simulink model "PIL_NO_RPI"  (R2021a)
settings: Solver=FixedStepAuto  StartTime=0.0  StopTime=50  FixedStep=0.001  RelTol=1e-3  EnableMultiTasking=on
undefined symbols (not defined in the file or in its folder): act_dmp, act_omega, Actuator, Aerodynamics, aMode, Autopilot, c_b_WGS, c_be, c_flat, c_grav, c_h_geop0, c_h_geope, c_pa0, c_pe, c_r0, c_rot, c_rsma, c_Tmp0, d_siB_0, d_siB_max, d_siB_min, dd_siB_max, dd_siB_min, DiscIntNeverNeededParam, e_pa, e_Tmp, fin_maxrate, flag_I_act_switch, flag_I_aero_switch, flag_I_flat, flag_I_gravity_switch, flag_I_rot, hcr, HIL_Data, JMMM_0, JMMM_e, JSPB_e, lat_0, lon_0, Mass_Props, mB_0, mM_0, mM_e, p, pBII_0, phi, pMPB, pNPB, propellant_kg, prp_FBPB, prp_mdot, prp_T, psi, pSPB, q, qEG_0, qIB_0, qIE_0, r, sgc ... (+28)
libraries: simulink x46, simulink_extras x10, aerolibcommonsys x4
(part 1 of 21)
settings Model: SimulationMode=external  CodeVerificationMode=processor-in-the-loop (pil)  ExtModeTrigDuration=10  Creator=m.hiepp  LastModifiedBy=benme
settings SolverCC: AlgebraicLoopSolver=TrustRegion  PositivePriorityOrder=on  AutoInsertRateTranBlk=on
settings DataIOCC: SignalLogging=off  ReturnWorkspaceOutputs=off
settings OptimizationCC: EnhancedBackFolding=on  PassReuseOutputArgsAs=Individual arguments  ZeroExternalMemoryAtStartup=off  ZeroInternalMemoryAtStartup=off  MaxStackSize=64  OptimizeBlockOrder=speed  DifferentSizesBufferReuse=on  OptimizationCustomize=off  EfficientTunableParamExpr=on
settings DebuggingCC: ParameterPrecisionLossMsg=none  ParameterTunabilityLossMsg=error  SFMachineParentedDataDiag=warning  UnderSpecifiedDimensionMsg=warning  ArithmeticOperatorsInVariantConditions=warning
settings HardwareCC: ProdBitPerPointer=32  ProdBitPerSizeT=32  ProdBitPerPtrDiffT=32  ProdLargestAtomicInteger=Long  ProdLargestAtomicFloat=Double  ProdWordSize=32  ProdLongLongMode=on  ProdHWDeviceType=ARM Compatible->ARM Cortex
settings SFSimCC: MATLABDynamicMemAlloc=off  CustomCodeUndefinedFunction=UseInterfaceOnly  SimTargetLang=C++
settings RTWCC: SystemTargetFile=ert.tlc  HardwareBoard=PX4 Pixhawk 2.1 (Cube)  TLCOptions="-aInlineSetEventsForThisBaseRateFcn=TLC_FALSE -aSuppressMultiTaskScheduler=TLC_FALSE  -aRateBasedStepFcn=0"  TemplateMakefile=ert_default_tmf  GenerateReport=on  Toolchain=GNU Tools for PX4 Autopilots  IncludeHyperlinkInReport=on  LaunchReport=on  PortableWordSizes=on  CreateSILPILBlock=PIL  TargetLang=C++  GenerateTraceInfo=on  GenerateTraceReport=on  GenerateTraceReportSl=on  GenerateTraceReportSf=on  GenerateTraceReportEml=on
settings CodeAppCC: ForceParamTrailComments=on  IgnoreCustomStorageClasses=off  MaxIdLength=95  OperatorAnnotations=on  SimulinkDataObjDesc=on  SFDataObjDesc=on  InsertBlockDesc=on
settings ERTTargetCC: SupportContinuousTime=on  ExtModeTransport=3  ExtModeStaticAlloc=on  ExtModeStaticAllocSize=1024  ExtModeMexFile=ext_xcp  ExtModeIntrfLevel=Level2 - Open

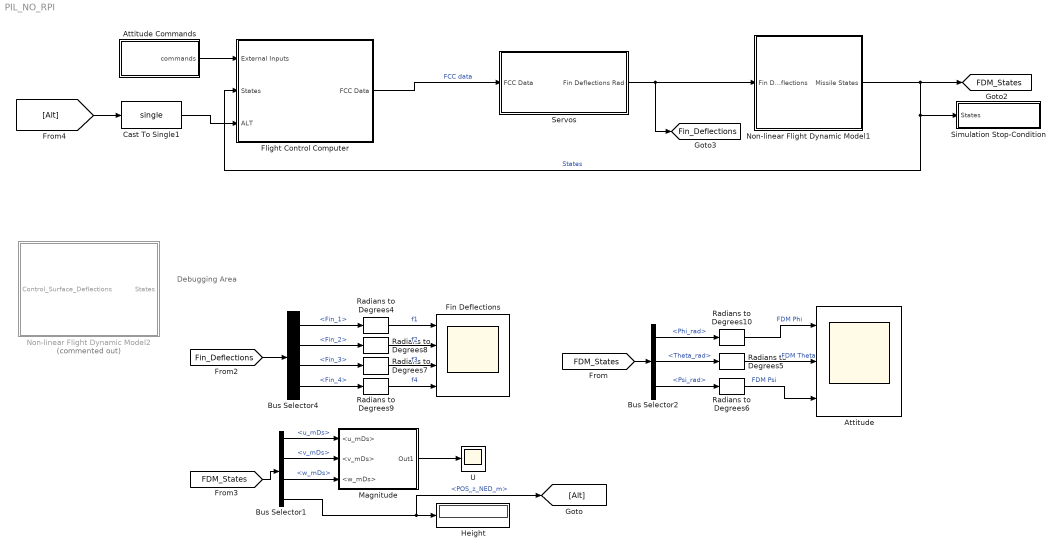
== system PIL_NO_RPI ==
  note: Debugging Area
  Attitude : Scope  NumInputPorts=3
  Attitude Commands : Subsystem
  Bus Selector1 : BusSelector  OutputSignals=Translation_States.u_mDs,Translation_States.v_mDs,Translation_States.w_mDs,POS_NED.POS_z_NED_m
  Bus Selector2 : BusSelector  OutputSignals=Attitude_States.ATT_Euler.Phi_rad,Attitude_States.ATT_Euler.Theta_rad,Attitude_States.ATT_Euler.Psi_rad
  Bus Selector4 : BusSelector  OutputSignals=Fin_1,Fin_2,Fin_3,Fin_4
  Cast To Single1 : DataTypeConversion  OutDataTypeStr=single
  Fin Deflections : Scope  NumInputPorts=4
  Flight Control Computer : Subsystem  VariantControl=VSS_FCC_REAL
  Height : Display
  Magnitude : Subsystem
  Non-linear Flight Dynamic Model1 : Subsystem  VariantControl=VSS_FDM_SOPH
      mask init:
      | load('generated_FDM_params')
  Non-linear Flight Dynamic Model2 : Subsystem  Commented=on  VariantControl=VSS_FDM_SOPH
      mask init:
      | load('generated_FDM_params')
  Radians to Degrees{4..10} (7 alike) : simulink_extras/Transformations/Radians to Degrees
  Servos : Subsystem  VariantControl=VSS_SERVOS_OFF
  Simulation Stop-Condition : Subsystem
  U : Scope
  tag scope: FDM_States=global, Fin_Deflections=global
  wires:
  Bus Selector2/3 -> Radians to Degrees6/1  "<Psi_rad>"
  Bus Selector4/2 -> Radians to Degrees8/1  "<Fin_2>"
  Bus Selector2/2 -> Radians to Degrees5/1  "<Theta_rad>"
  Radians to Degrees9/1 -> Fin Deflections/4  "f4"
  Radians to Degrees7/1 -> Fin Deflections/3  "f3"
  Radians to Degrees8/1 -> Fin Deflections/2  "f2"
  Bus Selector2/1 -> Radians to Degrees10/1  "<Phi_rad>"
  Servos/1(Fin Deflections Rad) -> Non-linear Flight Dynamic Model1/1(Fin Deflections), [Fin_Deflections]
  Bus Selector4/1 -> Radians to Degrees4/1  "<Fin_1>"
  [Fin_Deflections] -> Bus Selector4/1
  Attitude Commands/1(commands) -> Flight Control Computer/1(External Inputs)
  Radians to Degrees5/1 -> Attitude/2  "FDM Theta"
  [FDM_States] -> Bus Selector2/1
  Non-linear Flight Dynamic Model1/1(Missile States) -> Flight Control Computer/2(States), Simulation Stop-Condition/1(States), [FDM_States]  "States"
  Bus Selector4/3 -> Radians to Degrees7/1  "<Fin_3>"
  Radians to Degrees4/1 -> Fin Deflections/1  "f1"
  Radians to Degrees10/1 -> Attitude/1  "FDM Phi"
  Bus Selector4/4 -> Radians to Degrees9/1  "<Fin_4>"
  Radians to Degrees6/1 -> Attitude/3  "FDM Psi"
  Flight Control Computer/1(FCC Data) -> Servos/1(FCC Data)  "FCC data"
  [FDM_States] -> Bus Selector1/1
  Bus Selector1/4 -> [Alt], Height/1  "<POS_z_NED_m>"
  Bus Selector1/1 -> Magnitude/1(<u_mDs>)  "<u_mDs>"
  Bus Selector1/2 -> Magnitude/2(<v_mDs>)  "<v_mDs>"
  Bus Selector1/3 -> Magnitude/3(<w_mDs>)  "<w_mDs>"
  Magnitude/1(Out1) -> U/1
  Cast To Single1/1 -> Flight Control Computer/3("ALT ")
  [Alt] -> Cast To Single1/1

== system PIL_NO_RPI/Attitude Commands ==
  Bus Creator : BusCreator  Inputs=3
  Zero : Constant  Value=0  OutDataTypeStr=Inherit: Inherit via back propagation
  Zero1 : Constant  Value=0  OutDataTypeStr=Inherit: Inherit via back propagation
  Zero2 : Constant  Value=0  OutDataTypeStr=Inherit: Inherit via back propagation
  commands : Outport
  wires:
  Bus Creator/1 -> commands/1
  Zero/1 -> Bus Creator/3  "psi cmd rad"
  Zero1/1 -> Bus Creator/2  "theta cmd rad"
  Zero2/1 -> Bus Creator/1  "phi cmd rad"

== system PIL_NO_RPI/Flight Control Computer ==
  note: State Estimation:
      | 0 - use state variables calculated by FDM.
      | 1 - use or our own INS
  External Inputs : Inport
  States : Inport  Port=2
  "ALT " : Inport  Port=3
  Communication Delay - 7ms : Subsystem
  Communication Delay - 7ms1 : Subsystem
  Communication Delay - 7ms2 : Subsystem
  Constant4 : Constant  OutDataTypeStr=single
  Debug : Scope
  FCC Sync : Scope
  In Sync : Subsystem
  Pixhawk1 : Subsystem  TreatAsAtomicUnit=on  VariantControl=VSS_FCC_EMUL
  Recieve from Pixhawk : Subsystem
  Send to Pixhawk : Subsystem
  FCC Data : Outport
  wires:
  Constant4/1 -> Send to Pixhawk/3(Use FDM States)
  External Inputs/1 -> Send to Pixhawk/2(External_Inputs)
  States/1 -> Send to Pixhawk/1(States)
  Send to Pixhawk/1(Heartbeat Sent) -> In Sync/1(send)
  Recieve from Pixhawk/1(Heartbeat recieved1) -> In Sync/2(receive)  "receive"
  Recieve from Pixhawk/3(Other1) -> Debug/1
  In Sync/1(Heartbeat Sync) -> FCC Sync/1
  Communication Delay - 7ms2/1(Signal Recieved) -> Recieve from Pixhawk/1(data in1)
  Send to Pixhawk/2(data out) -> Communication Delay - 7ms/1(Signal Sent)
  "ALT "/1 -> Communication Delay - 7ms1/1(Signal Sent)
  Recieve from Pixhawk/2(fin_cmd_rad1) -> FCC Data/1
  Communication Delay - 7ms/1(Signal Recieved) -> Pixhawk1/1(Input Data)
  Communication Delay - 7ms1/1(Signal Recieved) -> Pixhawk1/2("ALT ")
  Pixhawk1/1(Output Data) -> Communication Delay - 7ms2/1(Signal Sent)

== system PIL_NO_RPI/Magnitude ==
  <u_mDs> : Inport
  <v_mDs> : Inport  Port=2
  <w_mDs> : Inport  Port=3
  Add1 : Sum  Inputs=+++
  Square Root1 : Sqrt  SaturateOnIntegerOverflow=on
  Square3 : Math  Operator=square  SaturateOnIntegerOverflow=on
  Square4 : Math  Operator=square  SaturateOnIntegerOverflow=on
  Square5 : Math  Operator=square  SaturateOnIntegerOverflow=on
  Out1 : Outport
  wires:
  Add1/1 -> Square Root1/1
  Square4/1 -> Add1/2
  Square5/1 -> Add1/3
  <u_mDs>/1 -> Square3/1
  Square Root1/1 -> Out1/1
  Square3/1 -> Add1/1
  <w_mDs>/1 -> Square5/1
  <v_mDs>/1 -> Square4/1

== system PIL_NO_RPI/Non-linear Flight Dynamic Model1 ==
  Fin Deflections : Inport
  Environment : Subsystem
  Extract States : Subsystem
  GRM_Airframe : Subsystem
      mask Display: image('$imagefile'); % Use "Edit Image" on toolstrip to change.
  Stop-Condition : Subsystem
  Subsystem1 : Subsystem  Commented=on
  Translate Fins : Subsystem
  Missile States : Outport  VectorParamsAs1DForOutWhenUnconnected=off
  wires:
  Fin Deflections/1 -> Translate Fins/1(Servo Deflections)
  Extract States/1(States) -> Missile States/1, Stop-Condition/1(States)  "States"
  Translate Fins/1(afinB) -> GRM_Airframe/1(siB_cmd)
  GRM_Airframe/1(airfr) -> Extract States/1(airfr_bus)
  Environment/1(env_glbl_bus) -> GRM_Airframe/2(T_sim_glbl)

== system PIL_NO_RPI/Non-linear Flight Dynamic Model2 ==
  note: This block is the work of Thomas. Should you have any questions, hes the guy to ask.
  Control_Surface_Deflections : Inport
  Extract Relevant States : Subsystem
  GRM_Airframe : Subsystem
      mask Display: image('$imagefile'); % Use "Edit Image" on toolstrip to change.
  Subsystem1 : Subsystem
  environment_global : Subsystem
  States : Outport  VectorParamsAs1DForOutWhenUnconnected=off
  wires:
  environment_global/1(env_glbl_bus) -> GRM_Airframe/2(T_sim_glbl)
  Subsystem1/1(afinB) -> GRM_Airframe/1(siB_cmd)
  Extract Relevant States/1(States) -> States/1
  Control_Surface_Deflections/1 -> Subsystem1/1(Servo Deflections)
  GRM_Airframe/1(airfr) -> Extract Relevant States/1(airfr_bus)

== system PIL_NO_RPI/Servos ==
  FCC Data : Inport
  Bus Creator : BusCreator  Inputs=4
  Bus Selector : BusSelector  OutputSignals=Fin_1_Cmd_rad,Fin_2_Cmd_rad,Fin_3_Cmd_rad,Fin_4_Cmd_rad
  Gain{,1..3} (4 alike) : Gain
  Transfer Fcn{1..4} (4 alike) : TransferFcn  Numerator=33770  Denominator=[1 395.7 33770]
  Fin Deflections Rad : Outport
  wires:
  FCC Data/1 -> Bus Selector/1
  Bus Selector/1 -> Transfer Fcn1/1  "<Fin_1_Cmd_rad>"
  Bus Selector/2 -> Transfer Fcn2/1  "<Fin_2_Cmd_rad>"
  Bus Selector/3 -> Transfer Fcn3/1  "<Fin_3_Cmd_rad>"
  Bus Selector/4 -> Transfer Fcn4/1  "<Fin_4_Cmd_rad>"
  Transfer Fcn1/1 -> Gain/1  "Fin_1"
  Transfer Fcn2/1 -> Gain1/1  "Fin_2"
  Transfer Fcn3/1 -> Gain2/1  "Fin_3"
  Transfer Fcn4/1 -> Gain3/1  "Fin_4"
  Bus Creator/1 -> Fin Deflections Rad/1
  Gain/1 -> Bus Creator/1  "Fin_1"
  Gain1/1 -> Bus Creator/2  "Fin_2"
  Gain2/1 -> Bus Creator/3  "Fin_3"
  Gain3/1 -> Bus Creator/4  "Fin_4"

== system PIL_NO_RPI/Simulation Stop-Condition ==
  note: Stops the simulation when the rocket hits the ground (Z~0)
  States : Inport
  Bus Selector1 : BusSelector  OutputSignals=POS_NED.POS_z_NED_m
  Compare To Constant : Subsystem  mask(Compare To Constant){relop=>=, const=-10*eps, OutDataTypeStr=boolean, ZeroCross=on}
      mask prompts: relop "Simulink:masks:Operator_MP"; const "Simulink:masks:ConstantValue_MP"; OutDataTypeStr "Simulink:masks:OutputDataType_MP"; ZeroCross "Simulink:masks:EnableZerocrossingDetection_MP"
      mask help: Simulink:masks:CompareToConstant_MD
      mask init:
      | blkName = gcb;
      | 
      | if strcmp(get_param(gcbh,'OutDataTypeStr'),'boolean')
      | 	setValue = 'boolean';
      | else
      | 	setValue = 'fixdt(0, 8)';
      | end
      | 
      | set_param([blkName,'/Compare'],'relop',relop, ...
      | 	'OutDataTypeStr', setValue, 'ZeroCross', ZeroCross);
      | 
      | str = [relop,' C']; %default
      | 
      | const_str = get_param(blkName, 'const');
      | const_val = str2num(const_str);
      | 
      | if isempty(const_val) %#ok<ST2NM>
      |     %Expression/Variable
      |     str = [relop, ' ', strtrim(const_str)];
      | else
      |     if length(const_val) == 1 
      |         if Simulink.data.isSupportedEnumClass(class(const_val))
      |             % Special Handling for Enumerations
      |             if Simulink.data.getEnumTypeInfo(class(const_val), 'AddClassNameToEnumNames')
      |                 str = [relop, ' ', strtrim(const_str)];
      |             else
      |                 str = [relop, ' ', char(const_val)];
      |             end
      |         elseif(isfloat(const_val) || isinteger(const_val) || islogical(const_val)) 
      |                 str = [relop, ' ', num2str(const_val)];
      |         end
      |     end
      | end
      mask TypeOptions relop: == | ~= | < | <= | >= | >
      mask TypeOptions OutDataTypeStr: Simulink:masks:uint8 | Simulink:masks:boolean
      mask Callback ZeroCross: sl('zeroCrossEnable', gcbh);
      mask Display: disp(str)
  Stop Simulation : Stop
  wires:
  Bus Selector1/1 -> Compare To Constant/1(u)  "<POS_z_NED_m>"
  States/1 -> Bus Selector1/1
  Compare To Constant/1(y) -> Stop Simulation/1

== system PIL_NO_RPI/Flight Control Computer/Communication Delay - 7ms ==
  Signal Sent : Inport
  Pulse Generator1 : DiscretePulseGenerator  PulseType=Time based  Period=0.01  PulseWidth=50
  Triggered Subsystem : Subsystem  TreatAsAtomicUnit=on
  Signal Recieved : Outport
  wires:
  Pulse Generator1/1 -> Triggered Subsystem/Trigger
  Signal Sent/1 -> Triggered Subsystem/1(In1)
  Triggered Subsystem/1(Out1) -> Signal Recieved/1

== system PIL_NO_RPI/Flight Control Computer/Communication Delay - 7ms1 ==
  Signal Sent : Inport
  Pulse Generator1 : DiscretePulseGenerator  PulseType=Time based  Period=0.01  PulseWidth=50
  Triggered Subsystem : Subsystem  TreatAsAtomicUnit=on
  Signal Recieved : Outport
  wires:
  Pulse Generator1/1 -> Triggered Subsystem/Trigger
  Signal Sent/1 -> Triggered Subsystem/1(In1)
  Triggered Subsystem/1(Out1) -> Signal Recieved/1

== system PIL_NO_RPI/Flight Control Computer/Communication Delay - 7ms2 ==
  Signal Sent : Inport
  Pulse Generator1 : DiscretePulseGenerator  PulseType=Time based  Period=0.01  PulseWidth=50
  Triggered Subsystem : Subsystem  TreatAsAtomicUnit=on
  Signal Recieved : Outport
  wires:
  Pulse Generator1/1 -> Triggered Subsystem/Trigger
  Signal Sent/1 -> Triggered Subsystem/1(In1)
  Triggered Subsystem/1(Out1) -> Signal Recieved/1

== system PIL_NO_RPI/Flight Control Computer/In Sync ==
  note: This block ensures the Pixhawk is connected and functioning correctly
  send : Inport
  receive : Inport  Port=2
  Cast To Single : DataTypeConversion  OutDataTypeStr=single
  Mux : Mux  Inputs=2
  Rate Transition : RateTransition  OutPortSampleTime=0.001
  Rate Transition1 : RateTransition  OutPortSampleTime=0.001
  Heartbeat Sync : Outport
  wires:
  receive/1 -> Rate Transition1/1  "receive"
  send/1 -> Rate Transition/1
  Rate Transition/1 -> Mux/1
  Rate Transition1/1 -> Cast To Single/1
  Mux/1 -> Heartbeat Sync/1
  Cast To Single/1 -> Mux/2

== system PIL_NO_RPI/Flight Control Computer/Pixhawk1 ==
  Input Data : Inport
  "ALT " : Inport  Port=2
  FCC Logic1 : Subsystem
  Send to HIL : Subsystem
  Terminator : Terminator
  Terminator1 : Terminator
  Zero1 : Constant  Value=-1  OutDataTypeStr=Inherit: Inherit via back propagation
  data2bus : Subsystem
  Output Data : Outport
  tag scope: heartbeatt=global
  wires:
  data2bus/2(FDM States) -> FCC Logic1/2(FDM States)
  data2bus/3(Heartbeat) -> [heartbeatt]
  [heartbeatt] -> Send to HIL/2(Heartbeat1)
  Zero1/1 -> Send to HIL/3(Debug Port1)
  FCC Logic1/1(Fin Deflections) -> Send to HIL/1(Fin Deflections1)
  data2bus/1(Ext. Commands) -> FCC Logic1/1(Ext. Commands)
  data2bus/4(FCC Enabled) -> Terminator/1
  data2bus/5(Use Sim States) -> Terminator1/1
  "ALT "/1 -> FCC Logic1/3(ALT)
  Send to HIL/1(Data Out) -> Output Data/1
  Input Data/1 -> data2bus/1(raw_data)

== system PIL_NO_RPI/Flight Control Computer/Recieve from Pixhawk ==
  data in1 : Inport
  Bus Creator2 : BusCreator  Inputs=4
  Cast To Double{18..23} (6 alike) : DataTypeConversion  OutDataTypeStr=double
  Demux1 : Demux  Outputs=6
  Heartbeat recieved1 : Outport
  fin_cmd_rad1 : Outport  Port=2  PortDimensions=4
  Other1 : Outport  Port=3
  wires:
  data in1/1 -> Demux1/1
  Demux1/3 -> Cast To Double20/1  "Fin_2_Cmd_rad"
  Cast To Double22/1 -> Bus Creator2/4  "Fin_4_Cmd_rad"
  Demux1/4 -> Cast To Double21/1  "Fin_3_Cmd_rad"
  Cast To Double18/1 -> Heartbeat recieved1/1
  Cast To Double19/1 -> Bus Creator2/1  "Fin_1_Cmd_rad"
  Cast To Double21/1 -> Bus Creator2/3  "Fin_3_Cmd_rad"
  Bus Creator2/1 -> fin_cmd_rad1/1
  Cast To Double20/1 -> Bus Creator2/2  "Fin_2_Cmd_rad"
  Demux1/2 -> Cast To Double19/1  "Fin_1_Cmd_rad"
  Demux1/1 -> Cast To Double18/1
  Demux1/5 -> Cast To Double22/1  "Fin_4_Cmd_rad"
  Cast To Double23/1 -> Other1/1  "gyroZ"
  Demux1/6 -> Cast To Double23/1

== system PIL_NO_RPI/Flight Control Computer/Send to Pixhawk ==
  States : Inport
  External_Inputs : Inport  Port=2
  Use FDM States : Inport  Port=3
  Bus Selector1 : BusSelector  OutputSignals=phi cmd rad
  Cast To Double{1..13} (13 alike) : DataTypeConversion  OutDataTypeStr=single
  HeartBeat : Subsystem
  Mux : Mux  Inputs=13
  One : Constant  OutDataTypeStr=Inherit: Inherit via back propagation
  Scope : Scope
  State Mixer : Subsystem
  Heartbeat Sent : Outport
  data out : Outport  Port=2
  wires:
  Cast To Double3/1 -> Mux/4
  Cast To Double1/1 -> Heartbeat Sent/1, Mux/2  "send"
  External_Inputs/1 -> Bus Selector1/1
  Cast To Double12/1 -> Mux/13
  Cast To Double10/1 -> Mux/11
  Cast To Double5/1 -> Mux/6
  Cast To Double2/1 -> Mux/3
  Cast To Double7/1 -> Mux/8
  Bus Selector1/1 -> Cast To Double12/1  "<phi cmd rad>"
  Cast To Double4/1 -> Mux/5
  Cast To Double8/1 -> Mux/9
  Cast To Double9/1 -> Mux/10
  Cast To Double6/1 -> Mux/7
  Cast To Double11/1 -> Mux/12
  States/1 -> State Mixer/1(States)
  State Mixer/1(Phi_rad) -> Cast To Double3/1
  State Mixer/2(Theta_rad) -> Cast To Double4/1
  State Mixer/3(Psi_rad) -> Cast To Double5/1
  State Mixer/4(p_radDs) -> Cast To Double6/1
  State Mixer/5(q_radDs) -> Cast To Double7/1
  State Mixer/6(r_radDs) -> Cast To Double8/1
  State Mixer/7(u_mDs) -> Cast To Double9/1
  State Mixer/8(v_mDs) -> Cast To Double10/1
  State Mixer/9(w_mDs) -> Cast To Double11/1
  Cast To Double13/1 -> Mux/1  "send"
  One/1 -> Cast To Double13/1
  Use FDM States/1 -> Cast To Double2/1
  Mux/1 -> Scope/1, data out/1  "send"
  HeartBeat/1(Out1) -> Cast To Double1/1

== system PIL_NO_RPI/Non-linear Flight Dynamic Model1/Environment ==
  Add : Sum  Inputs=-+
  Bus Creator1 : BusCreator  Inputs=5
  Clock : Clock
  Constant6 : Constant  Value=T_sim_lnch
  Enabled Subsystem1 : Subsystem  TreatAsAtomicUnit=on
  From10 : From  Commented=on  GotoTag=HIL_Ready  TagVisibility=global
  Memory : Memory
  NOT : Logic  Operator=NOT  IconShape=distinctive  AllPortsSameDT=off  OutDataTypeStr=boolean
  atm_dynamic : Subsystem
  deviation_Tmp : Constant  Value=e_Tmp
  deviation_pa_QFH : Constant  Value=e_pa
  env_glbl_bus : Outport
  wires:
  atm_dynamic/1(vWEG) -> Bus Creator1/3
  Bus Creator1/1 -> env_glbl_bus/1  "env_glbl_bus"
  Clock/1 -> Add/2
  Constant6/1 -> Bus Creator1/2  "T_sim_lnch"
  deviation_pa_QFH/1 -> Bus Creator1/5  "e_pa"
  deviation_Tmp/1 -> Bus Creator1/4  "e_Tmp"
  From10/1 -> ?
  Add/1 -> Bus Creator1/1  "T_sim_glbl"
  Enabled Subsystem1/1(CalibrationTime) -> Add/1, NOT/1
  Memory/1 -> Enabled Subsystem1/Enable
  NOT/1 -> Memory/1

== system PIL_NO_RPI/Non-linear Flight Dynamic Model1/Extract States ==
  airfr_bus : Inport
  Assemble_States_Bus1 : Subsystem
  Bus Selector1 : BusSelector  OutputSignals=flight_dyn_bus.vBIB,flight_dyn_bus.wBIB,flight_dyn_bus.aBIB,flight_dyn_bus.d_wBIB,flight_dyn_bus.qIB,flight_dyn_bus.pBII,flight_dyn_bus.vBII
  MATLAB Function1 : MATLAB Function  TreatAsAtomicUnit=on
  quaternion_to_euler_angles1 : Subsystem
      mask help: transforms quaternions to Euler angles (roll, pitch, yaw)
      mask Help:
      | Name:
      | 
      |     quaternion_to_euler_angles
      | 
      | Description:
      | 
      |     This block implements the transformation of a quaternion into the
      |     corresponding Euler angles (zyx-sequence, roll, pitch, yaw).
      | 
      | Inputs  [size] [data type] [unit]:
      | 
      |     quaternion  [4] [double] [-]
      | 
      | Outputs  [size] [data type] [unit]:
      | 
      |     roll angle phi  [1] [double] [rad]
      |     pitch angle theta  [1] [double] [rad]
      |     yaw angle psi  [1] [double] [rad]
      mask Display:
      | %disp (' q --> (Phi,Theta,Psi) [rad]')
      | disp('q \rightarrow eu(\Phi;\Theta;\Psi)','texmode','on')
  States : Outport
  wires:
  Bus Selector1/6 -> Assemble_States_Bus1/6(POS_NED)  "<pBII>"
  quaternion_to_euler_angles1/1(eulx) -> Assemble_States_Bus1/5(Attitude_States)  "from Quat"
  MATLAB Function1/1(q_conj) -> quaternion_to_euler_angles1/1(q)
  Bus Selector1/5 -> MATLAB Function1/1(q)  "<qIB>"
  airfr_bus/1 -> Bus Selector1/1
  Bus Selector1/1 -> Assemble_States_Bus1/1(Translation_States)  "<vBIB>"
  Bus Selector1/2 -> Assemble_States_Bus1/2(Rotation_States)  "<wBIB>"
  Bus Selector1/4 -> Assemble_States_Bus1/4(Rotation_States_Dot)  "<d_wBIB>"
  Bus Selector1/3 -> Assemble_States_Bus1/3(Translation_States_Dot)  "<aBIB>"
  Assemble_States_Bus1/1(States) -> States/1
  Bus Selector1/7 -> Assemble_States_Bus1/7(POS_NED_dot)  "<vBII>"

== system PIL_NO_RPI/Non-linear Flight Dynamic Model1/GRM_Airframe ==
  siB_cmd : Inport
  T_sim_glbl : Inport  Port=2
  Bus Creator : BusCreator  Inputs=9
  aerodynamics : Subsystem
  environment : Subsystem
  fin_actuators : Subsystem
  forces_moments : Subsystem
  gravity : Subsystem
  input : Subsystem
  motion_kinematics : Subsystem
  propulsion : Subsystem
  rb_eom : Subsystem
  stream_flow : Subsystem
  weight_and_balance : Subsystem
  airfr : Outport  VectorParamsAs1DForOutWhenUnconnected=off
  wires:
  forces_moments/1(for_mom_bus) -> rb_eom/2(for_mom)
  [env] -> Bus Creator/9
  [fin] -> Bus Creator/7
  [motion_kin] -> Bus Creator/6
  [env_glbl] -> aerodynamics/4(env_glbl)
  aerodynamics/1(aero) -> forces_moments/1(aero), [aero]
  [motion_kin] -> rb_eom/1(mot_kin)
  weight_and_balance/1(wab) -> rb_eom/3(wab), gravity/2(wab), [wab], propulsion/2(wab)
  [wab] -> aerodynamics/3(wab)
  [str_flow] -> Bus Creator/5
  [motion_kin] -> forces_moments/2(motion_kin)
  motion_kinematics/1(motion_kin) -> stream_flow/2(motion_kin), [motion_kin]
  [grav] -> Bus Creator/3
  Bus Creator/1 -> airfr/1  "airfr_bus"
  [aero] -> Bus Creator/4
  environment/1(env) -> [env], stream_flow/3(env), gravity/1(env)
  [prp] -> forces_moments/4(prp)
  [prp] -> Bus Creator/8
  stream_flow/1(str_flow) -> [str_flow], aerodynamics/1(str_flow)
  input/1(cmd_bus) -> fin_actuators/1(cmd)
  [wab] -> Bus Creator/2
  gravity/1(grav) -> [grav], forces_moments/3(grav)
  T_sim_glbl/1 -> [env_glbl], environment/2(env_glbl), weight_and_balance/1(env_glb), propulsion/1(env_glbl)
  siB_cmd/1 -> input/1(siB_cmd)
  rb_eom/1(flight_dyn) -> environment/1(flight_dyn), motion_kinematics/1(flight_dyn), stream_flow/1(flight_dyn), Bus Creator/1
  fin_actuators/1(fin) -> [fin], aerodynamics/2(fin)
  propulsion/1(prp) -> [prp]

== system PIL_NO_RPI/Non-linear Flight Dynamic Model1/Stop-Condition ==
  States : Inport
  AND : Logic  Inputs=3  IconShape=distinctive  AllPortsSameDT=off  OutDataTypeStr=boolean
  Bus Selector1 : BusSelector  OutputSignals=POS_NED.POS_z_NED_m,POS_NED_dot.POS_z_NED_dot_m
  Compare To Constant : Subsystem  mask(Compare To Constant){relop=>, const=-700, OutDataTypeStr=boolean, ZeroCross=on}
      mask prompts: relop "Simulink:masks:Operator_MP"; const "Simulink:masks:ConstantValue_MP"; OutDataTypeStr "Simulink:masks:OutputDataType_MP"; ZeroCross "Simulink:masks:EnableZerocrossingDetection_MP"
      mask help: Simulink:masks:CompareToConstant_MD
      mask init: same as PIL_NO_RPI/Simulation Stop-Condition/Compare To Constant
      mask TypeOptions relop: == | ~= | < | <= | >= | >
      mask TypeOptions OutDataTypeStr: Simulink:masks:uint8 | Simulink:masks:boolean
      mask Callback ZeroCross: sl('zeroCrossEnable', gcbh);
      mask Display: disp(str)
  Compare To Constant1 : Subsystem  mask(Compare To Constant){relop=>, const=0, OutDataTypeStr=boolean, ZeroCross=on}
      mask prompts: relop "Simulink:masks:Operator_MP"; const "Simulink:masks:ConstantValue_MP"; OutDataTypeStr "Simulink:masks:OutputDataType_MP"; ZeroCross "Simulink:masks:EnableZerocrossingDetection_MP"
      mask help: Simulink:masks:CompareToConstant_MD
      mask init: same as PIL_NO_RPI/Simulation Stop-Condition/Compare To Constant
      mask TypeOptions relop: == | ~= | < | <= | >= | >
      mask TypeOptions OutDataTypeStr: Simulink:masks:uint8 | Simulink:masks:boolean
      mask Callback ZeroCross: sl('zeroCrossEnable', gcbh);
      mask Display: disp(str)
  From4 : From  Commented=on  GotoTag=HIL_Ready  TagVisibility=global
  Stop Simulation : Stop
  wires:
  Bus Selector1/1 -> Compare To Constant/1(u)  "<POS_z_NED_m>"
  States/1 -> Bus Selector1/1
  Compare To Constant/1(y) -> AND/2
  AND/1 -> Stop Simulation/1
  From4/1 -> AND/1
  Bus Selector1/2 -> Compare To Constant1/1(u)  "<POS_z_NED_dot_m>"
  Compare To Constant1/1(y) -> AND/3

== system PIL_NO_RPI/Non-linear Flight Dynamic Model1/Subsystem1 ==
  Control Surface Deflections : Inport
  Envoronment : Inport  Port=2
  Enable : EnablePort
  Extract States : Subsystem
  Fin Deflections : Subsystem
  GRM_Airframe : Subsystem
      mask Display: image('$imagefile'); % Use "Edit Image" on toolstrip to change.
  Missile States : Outport
  wires:
  GRM_Airframe/1(airfr) -> Extract States/1(airfr_bus)
  Control Surface Deflections/1 -> Fin Deflections/1(Servo Deflections)
  Envoronment/1 -> GRM_Airframe/2(T_sim_glbl)
  Extract States/1(States) -> Missile States/1
  Fin Deflections/1(afinB) -> GRM_Airframe/1(siB_cmd)

== system PIL_NO_RPI/Non-linear Flight Dynamic Model1/Translate Fins ==
  Servo Deflections : Inport
  Add : Sum
  Bus Selector : BusSelector  OutputSignals=Fin_1,Fin_2,Fin_3,Fin_4
  Constant1 : Constant  Value=unc_fin_def_roll
  Constant2 : Constant  Value=unc_fin_def_pitch
  Constant3 : Constant  Value=unc_fin_def_yaw
  Degrees to Radians : Subsystem  mask(DegreesToRadians){}
      mask help: SimulinkBlocks:simulink_extras:DegreesToRadians_MD
      mask Help: web([docroot '/simulink/ref_extras/degreestoradians.html'])
      mask Display: disp('D2R')
  Degrees to Radians1 : Subsystem  mask(DegreesToRadians){}
      mask help: SimulinkBlocks:simulink_extras:DegreesToRadians_MD
      mask Help: web([docroot '/simulink/ref_extras/degreestoradians.html'])
      mask Display: disp('D2R')
  Degrees to Radians2 : Subsystem  mask(DegreesToRadians){}
      mask help: SimulinkBlocks:simulink_extras:DegreesToRadians_MD
      mask Help: web([docroot '/simulink/ref_extras/degreestoradians.html'])
      mask Display: disp('D2R')
  Vector Concatenate : Concatenate  NumInputs=4
  Vector Concatenate1 : Concatenate  NumInputs=3
  control_allocation : Subsystem
  afinB : Outport
  wires:
  Degrees to Radians2/1(Radians out) -> Vector Concatenate1/3
  Vector Concatenate1/1 -> control_allocation/1(fin_cmd)  "fin_cmd"
  Constant1/1 -> Degrees to Radians/1(Degrees in)  "xi_cmd"
  Degrees to Radians1/1(Radians out) -> Vector Concatenate1/2
  Degrees to Radians/1(Radians out) -> Vector Concatenate1/1
  Constant3/1 -> Degrees to Radians2/1(Degrees in)  "ze_cmd"
  Constant2/1 -> Degrees to Radians1/1(Degrees in)  "et_cmd"
  Bus Selector/2 -> Vector Concatenate/2  "<Fin_2>"
  Servo Deflections/1 -> Bus Selector/1
  Bus Selector/1 -> Vector Concatenate/1  "<Fin_1>"
  Bus Selector/4 -> Vector Concatenate/4  "<Fin_4>"
  Vector Concatenate/1 -> Add/1
  Bus Selector/3 -> Vector Concatenate/3  "<Fin_3>"
  control_allocation/1(siB_cmd) -> Add/2
  Add/1 -> afinB/1  "siB_cmd"

== system PIL_NO_RPI/Non-linear Flight Dynamic Model2/Extract Relevant States ==
  airfr_bus : Inport
  Assemble_States_Bus1 : Subsystem
  Bus Selector1 : BusSelector  OutputSignals=flight_dyn_bus.vBIB,flight_dyn_bus.wBIB,flight_dyn_bus.aBIB,flight_dyn_bus.d_wBIB,flight_dyn_bus.qIB,flight_dyn_bus.pBII,flight_dyn_bus.vBII
  MATLAB Function1 : MATLAB Function  TreatAsAtomicUnit=on
  Terminator : Terminator
  quaternion_to_euler_angles1 : Subsystem
      mask help: transforms quaternions to Euler angles (roll, pitch, yaw)
      mask Help:
      | Name:
      | 
      |     quaternion_to_euler_angles
      | 
      | Description:
      | 
      |     This block implements the transformation of a quaternion into the
      |     corresponding Euler angles (zyx-sequence, roll, pitch, yaw).
      | 
      | Inputs  [size] [data type] [unit]:
      | 
      |     quaternion  [4] [double] [-]
      | 
      | Outputs  [size] [data type] [unit]:
      | 
      |     roll angle phi  [1] [double] [rad]
      |     pitch angle theta  [1] [double] [rad]
      |     yaw angle psi  [1] [double] [rad]
      mask Display:
      | %disp (' q --> (Phi,Theta,Psi) [rad]')
      | disp('q \rightarrow eu(\Phi;\Theta;\Psi)','texmode','on')
  States : Outport
  wires:
  Bus Selector1/6 -> Assemble_States_Bus1/6(POS_NED)  "<pBII>"
  quaternion_to_euler_angles1/1(eulx) -> Assemble_States_Bus1/5(Attitude_States)  "from Quat"
  MATLAB Function1/1(q_conj) -> quaternion_to_euler_angles1/1(q)
  Bus Selector1/5 -> MATLAB Function1/1(q)  "<qIB>"
  airfr_bus/1 -> Bus Selector1/1
  Bus Selector1/1 -> Assemble_States_Bus1/1(Translation_States)  "<vBIB>"
  Bus Selector1/2 -> Assemble_States_Bus1/2(Rotation_States)  "<wBIB>"
  Bus Selector1/4 -> Assemble_States_Bus1/4(Rotation_States_Dot)  "<d_wBIB>"
  Bus Selector1/3 -> Assemble_States_Bus1/3(Translation_States_Dot)  "<aBIB>"
  Assemble_States_Bus1/1(States) -> States/1
  Bus Selector1/7 -> Terminator/1  "<vBII>"

== system PIL_NO_RPI/Non-linear Flight Dynamic Model2/GRM_Airframe ==
  siB_cmd : Inport
  T_sim_glbl : Inport  Port=2
  Bus Creator : BusCreator  Inputs=9
  aerodynamics : Subsystem
  environment : Subsystem
  fin_actuators : Subsystem
  forces_moments : Subsystem
  gravity : Subsystem
  input : Subsystem
  motion_kinematics : Subsystem
  propulsion : Subsystem
  rb_eom : Subsystem
  stream_flow : Subsystem
  weight_and_balance : Subsystem
  airfr : Outport  VectorParamsAs1DForOutWhenUnconnected=off
  wires:
  propulsion/1(prp) -> [prp]
  fin_actuators/1(fin) -> aerodynamics/2(fin), [fin]
  rb_eom/1(flight_dyn) -> Bus Creator/1, stream_flow/1(flight_dyn), motion_kinematics/1(flight_dyn), environment/1(flight_dyn)
  siB_cmd/1 -> input/1(siB_cmd)
  T_sim_glbl/1 -> propulsion/1(env_glbl), weight_and_balance/1(env_glb), environment/2(env_glbl), [env_glbl]
  gravity/1(grav) -> forces_moments/3(grav), [grav]
  [wab] -> Bus Creator/2
  input/1(cmd_bus) -> fin_actuators/1(cmd)
  stream_flow/1(str_flow) -> aerodynamics/1(str_flow), [str_flow]
  [prp] -> Bus Creator/8
  [prp] -> forces_moments/4(prp)
  environment/1(env) -> gravity/1(env), stream_flow/3(env), [env]
  [aero] -> Bus Creator/4
  Bus Creator/1 -> airfr/1  "airfr_bus"
  [grav] -> Bus Creator/3
  motion_kinematics/1(motion_kin) -> [motion_kin], stream_flow/2(motion_kin)
  [motion_kin] -> forces_moments/2(motion_kin)
  [str_flow] -> Bus Creator/5
  [wab] -> aerodynamics/3(wab)
  weight_and_balance/1(wab) -> propulsion/2(wab), [wab], gravity/2(wab), rb_eom/3(wab)
  [motion_kin] -> rb_eom/1(mot_kin)
  aerodynamics/1(aero) -> [aero], forces_moments/1(aero)
  [env_glbl] -> aerodynamics/4(env_glbl)
  [motion_kin] -> Bus Creator/6
  [fin] -> Bus Creator/7
  [env] -> Bus Creator/9
  forces_moments/1(for_mom_bus) -> rb_eom/2(for_mom)

== system PIL_NO_RPI/Non-linear Flight Dynamic Model2/Subsystem1 ==
  Servo Deflections : Inport
  Add : Sum
  Bus Selector : BusSelector  OutputSignals=Fin_1,Fin_2,Fin_3,Fin_4
  Constant1 : Constant  Value=unc_fin_def_roll
  Constant2 : Constant  Value=unc_fin_def_pitch
  Constant3 : Constant  Value=unc_fin_def_yaw
  Degrees to Radians : Subsystem  mask(DegreesToRadians){}
      mask help: SimulinkBlocks:simulink_extras:DegreesToRadians_MD
      mask Help: web([docroot '/simulink/ref_extras/degreestoradians.html'])
      mask Display: disp('D2R')
  Degrees to Radians1 : Subsystem  mask(DegreesToRadians){}
      mask help: SimulinkBlocks:simulink_extras:DegreesToRadians_MD
      mask Help: web([docroot '/simulink/ref_extras/degreestoradians.html'])
      mask Display: disp('D2R')
  Degrees to Radians2 : Subsystem  mask(DegreesToRadians){}
      mask help: SimulinkBlocks:simulink_extras:DegreesToRadians_MD
      mask Help: web([docroot '/simulink/ref_extras/degreestoradians.html'])
      mask Display: disp('D2R')
  Vector Concatenate : Concatenate  NumInputs=4
  Vector Concatenate1 : Concatenate  NumInputs=3
  control_allocation : Subsystem
  afinB : Outport
  wires:
  Degrees to Radians2/1(Radians out) -> Vector Concatenate1/3
  Vector Concatenate1/1 -> control_allocation/1(fin_cmd)  "fin_cmd"
  Constant1/1 -> Degrees to Radians/1(Degrees in)  "xi_cmd"
  Degrees to Radians1/1(Radians out) -> Vector Concatenate1/2
  Degrees to Radians/1(Radians out) -> Vector Concatenate1/1
  Constant3/1 -> Degrees to Radians2/1(Degrees in)  "ze_cmd"
  Constant2/1 -> Degrees to Radians1/1(Degrees in)  "et_cmd"
  Bus Selector/2 -> Vector Concatenate/2  "<Fin_2>"
  Servo Deflections/1 -> Bus Selector/1
  Bus Selector/1 -> Vector Concatenate/1  "<Fin_1>"
  Bus Selector/4 -> Vector Concatenate/4  "<Fin_4>"
  Vector Concatenate/1 -> Add/1
  Bus Selector/3 -> Vector Concatenate/3  "<Fin_3>"
  control_allocation/1(siB_cmd) -> Add/2
  Add/1 -> afinB/1  "siB_cmd"

== system PIL_NO_RPI/Non-linear Flight Dynamic Model2/environment_global ==
  Bus Creator1 : BusCreator  Inputs=5
  Clock : Clock
  Constant6 : Constant  Value=T_sim_lnch
  atm_dynamic : Subsystem
  deviation_Tmp : Constant  Value=e_Tmp
  deviation_pa_QFH : Constant  Value=e_pa
  env_glbl_bus : Outport
  wires:
  atm_dynamic/1(vWEG) -> Bus Creator1/3
  Bus Creator1/1 -> env_glbl_bus/1  "env_glbl_bus"
  Constant6/1 -> Bus Creator1/2  "T_sim_lnch"
  deviation_pa_QFH/1 -> Bus Creator1/5  "e_pa"
  deviation_Tmp/1 -> Bus Creator1/4  "e_Tmp"
  Clock/1 -> Bus Creator1/1  "T_sim_glbl"

== system PIL_NO_RPI/Simulation Stop-Condition/Compare To Constant ==
  u : Inport
  Compare : RelationalOperator  OutDataTypeStr=boolean  RndMeth=Nearest  InputSameDT=on
  Constant : Constant  DisableCoverage=on  Value=const  OutDataTypeStr=Inherit: Inherit via back propagation
  y : Outport
  wires:
  u/1 -> Compare/1
  Constant/1 -> Compare/2
  Compare/1 -> y/1

== system PIL_NO_RPI/Flight Control Computer/Communication Delay - 7ms/Triggered Subsystem ==
  In1 : Inport
  Trigger : TriggerPort  VariantControl=Variant
  Out1 : Outport
  wires:
  In1/1 -> Out1/1

== system PIL_NO_RPI/Flight Control Computer/Communication Delay - 7ms1/Triggered Subsystem ==
  In1 : Inport
  Trigger : TriggerPort  VariantControl=Variant
  Out1 : Outport
  wires:
  In1/1 -> Out1/1

== system PIL_NO_RPI/Flight Control Computer/Communication Delay - 7ms2/Triggered Subsystem ==
  In1 : Inport
  Trigger : TriggerPort  VariantControl=Variant
  Out1 : Outport
  wires:
  In1/1 -> Out1/1

== system PIL_NO_RPI/Flight Control Computer/Pixhawk1/FCC Logic1 ==
  Ext. Commands : Inport
  FDM States : Inport  Port=2
  ALT : Inport  Port=3
  Control : Subsystem
  Fin Allocation1 : Subsystem
  Fin Allocation2 : Subsystem  Commented=on
  variable switch : Subsystem
  Fin Deflections : Outport
  wires:
  Fin Allocation1/1(Fin Cmd) -> Fin Deflections/1
  Control/1(Attitude_Commands) -> Fin Allocation1/1(Attitude Cmd)  "ATT_Cmd"
  Ext. Commands/1 -> Control/1(cmd)
  variable switch/1(State Bus) -> Control/2(states)
  FDM States/1 -> variable switch/1(Simulation States)
  ALT/1 -> Control/3(ALT)

== system PIL_NO_RPI/Flight Control Computer/Pixhawk1/Send to HIL ==
  Fin Deflections1 : Inport
  Heartbeat1 : Inport  Port=2
  Debug Port1 : Inport  Port=3
  Cast To Single : DataTypeConversion  OutDataTypeStr=single
  Cast To Single3 : DataTypeConversion  OutDataTypeStr=single
  Cast To Single4 : DataTypeConversion  OutDataTypeStr=single
  Demux1 : Demux
  Vector Concatenate1 : Concatenate  NumInputs=6
  control_allocation : Subsystem
  Data Out : Outport
  wires:
  Cast To Single/1 -> Data Out/1
  Heartbeat1/1 -> Vector Concatenate1/1
  control_allocation/1(siB_cmd) -> Cast To Single4/1
  Fin Deflections1/1 -> Cast To Single3/1
  Cast To Single3/1 -> control_allocation/1(fin_cmd)
  Cast To Single4/1 -> Demux1/1
  Demux1/1 -> Vector Concatenate1/2  "siB_cmd_1"
  Demux1/2 -> Vector Concatenate1/3  "siB_cmd_2"
  Demux1/3 -> Vector Concatenate1/4  "siB_cmd_3"
  Demux1/4 -> Vector Concatenate1/5  "siB_cmd_4"
  Debug Port1/1 -> Vector Concatenate1/6
  Vector Concatenate1/1 -> Cast To Single/1

== system PIL_NO_RPI/Flight Control Computer/Pixhawk1/data2bus ==
  raw_data : Inport  OutDataTypeStr=single
  100Hz Reset : Subsystem
  Bus Creator : BusCreator  Inputs=9
  Bus Creator1 : BusCreator  Inputs=1
  Demux : Demux  Outputs=13
  Ext. Commands : Outport  OutDataTypeStr=single
  FDM States : Outport  Port=2  OutDataTypeStr=single
  Heartbeat : Outport  Port=3
  FCC Enabled : Outport  Port=4
  Use Sim States : Outport  Port=5
  tag scope: rst=global
  wires:
  Demux/10 -> Bus Creator/7  "u"
  Demux/3 -> Use Sim States/1  "Use Sim States"
  Demux/8 -> Bus Creator/5  "q"
  Demux/4 -> Bus Creator/1  "phi"
  Demux/5 -> Bus Creator/2  "theta"
  Demux/7 -> Bus Creator/4  "p"
  Demux/9 -> Bus Creator/6  "r"
  Demux/6 -> Bus Creator/3  "psi"
  Demux/13 -> Bus Creator1/1  "phi_cmd"
  Demux/12 -> Bus Creator/9  "w"
  Demux/11 -> Bus Creator/8  "v"
  raw_data/1 -> Demux/1
  Bus Creator/1 -> FDM States/1
  Bus Creator1/1 -> Ext. Commands/1
  Demux/1 -> FCC Enabled/1  "EnableFCC"
  100Hz Reset/1(RST) -> [rst]
  Demux/2 -> 100Hz Reset/1(Heartbeat), Heartbeat/1  "Hearbeat"

== system PIL_NO_RPI/Flight Control Computer/Send to Pixhawk/HeartBeat ==
  note: Starting the heartbeat at negative values prevents unwanted FCC behaviour on startup
  Cast To Double14 : DataTypeConversion  OutDataTypeStr=single
  Heartbeat : simulink/Sources/Counter Free-Running  NumBits=16  tsamp=-1
  Subtract : Sum  Inputs=+-
  Zero : Constant  Value=1000  OutDataTypeStr=Inherit: Inherit via back propagation
  Out1 : Outport
  wires:
  Heartbeat/1 -> Cast To Double14/1
  Zero/1 -> Subtract/2
  Cast To Double14/1 -> Subtract/1  "send"
  Subtract/1 -> Out1/1

== system PIL_NO_RPI/Flight Control Computer/Send to Pixhawk/State Mixer ==
  States : Inport
  Bus Selector : BusSelector  OutputSignals=Attitude_States.ATT_Euler.Phi_rad,Attitude_States.ATT_Euler.Theta_rad,Attitude_States.ATT_Euler.Psi_rad,Rotation_States.p_radDs,Rotation_States.q_radDs,Rotation_States.r_radDs,Translation_States.u_mDs,Translation_States.v_mDs,Translation_States.w_mDs
  Phi_rad : Outport
  Theta_rad : Outport  Port=2
  Psi_rad : Outport  Port=3
  p_radDs : Outport  Port=4
  q_radDs : Outport  Port=5
  r_radDs : Outport  Port=6
  u_mDs : Outport  Port=7
  v_mDs : Outport  Port=8
  w_mDs : Outport  Port=9
  wires:
  Bus Selector/3 -> Psi_rad/1  "<Psi_rad>"
  Bus Selector/9 -> w_mDs/1  "<w_mDs>"
  Bus Selector/1 -> Phi_rad/1  "<Phi_rad>"
  Bus Selector/5 -> q_radDs/1  "<q_radDs>"
  Bus Selector/7 -> u_mDs/1  "<u_mDs>"
  Bus Selector/6 -> r_radDs/1  "<r_radDs>"
  Bus Selector/2 -> Theta_rad/1  "<Theta_rad>"
  States/1 -> Bus Selector/1
  Bus Selector/8 -> v_mDs/1  "<v_mDs>"
  Bus Selector/4 -> p_radDs/1  "<p_radDs>"

== system PIL_NO_RPI/Non-linear Flight Dynamic Model1/Environment/Enabled Subsystem1 ==
  Enable : EnablePort
  Digital Clock : DigitalClock  SampleTime=-1
  CalibrationTime : Outport  InitialOutput=0
  wires:
  Digital Clock/1 -> CalibrationTime/1

== system PIL_NO_RPI/Non-linear Flight Dynamic Model1/Environment/atm_dynamic ==
  Add : Sum
  Add1 : Sum
  Bus Creator : BusCreator  Inputs=1
  Constant1 : Constant  Value=0
  Vector Concatenate : Concatenate  NumInputs=3
  course_angle_uncertainty : Constant  Value=0
  course_angle_wind : Constant  Value=0
  trafo_around_z_axis : Subsystem  mask(Transformation um z-Achse){}
      mask help: Dieser Block transformiert einen Vektor vec1 durch eine Drehung des Referenzkoordinatensystems um die z-Achse und um den Winkel gamma (in rad) in den Vektor vec2
      mask Help:
      | Name:
      | 
      |    trafo_around_z_axis
      | 
      | Beschreibung:
      | 
      |    Dieser Block transformiert einen Vektor vec1 durch eine Drehung des
      |    Referenzkoordinatensystems um die z-Achse und um den Winkel gamma
      |    (in rad) in den Vektor vec2
      | 
      | Inputs   [dimension]  [data type] [unit]:
      | 
      |     vec1    [3] [double] [-]
      |     gamma   [1] [double] [rad]
      | 
      | Outputs  [dimension]  [data type] [unit]:
      | 
      |     vec2  [3] [double] [-]
  vWW : Constant  Value=0
  vWW_uncertainty : Constant  Value=0
  vWEG : Outport  VectorParamsAs1DForOutWhenUnconnected=off
  wires:
  Bus Creator/1 -> vWEG/1  "atm_dyn_bus"
  trafo_around_z_axis/1(vec2) -> Bus Creator/1  "vWEG"
  Add1/1 -> Vector Concatenate/1
  course_angle_uncertainty/1 -> Add/2
  Constant1/1 -> Vector Concatenate/2, Vector Concatenate/3
  vWW/1 -> Add1/2
  Vector Concatenate/1 -> trafo_around_z_axis/1(vec1)
  Add/1 -> trafo_around_z_axis/2(gamma)
  vWW_uncertainty/1 -> Add1/1
  course_angle_wind/1 -> Add/1
